simulink library "TOWER_MASTER"  (Simulink 8.8)
settings: Solver=ode45  StartTime=0.0  StopTime=10.0  RelTol=1e-3  EnableMultiTasking=on
undefined symbols (not defined in the file): AC, AC2THRESHOLD, BF_WD_MASTER, GAS_WD_MASTER, GASAC, SIXOSEM_F_WD_AC_MASTER
libraries: cdsEpicsOut x163, cdsFilt x111, cdsTP x68, cdsFiltCtrl x56, cdsEpicsIn x47, cdsMuxMatrix x14, cdsRms x14, TOWER_MASTER x11, STATE_BIO_MASTER x8, cdsEpicsBinIn x6, cdsFunctionCall x4, VIS_LIB x2
(part 16 of 19)

== system TOWER_MASTER/common_blocks/GASMASTER/SEISFF ==
  note: 1 (one) if GOOD
      | 0 (zero) if BAD
  note: Each DAMP filter output bitword is
      | compared against a known good state.
      | If equal to good state, then a 1 is output
      | and multiplied into the product. So, if any DOF
      | is not in its good state, the whole product is 0.
  SEIS_In : Inport
  GAS : cdsFiltCtrl/IIR FM with control  Tag=cdsFiltCtrl  Description=|
      | cdsFiltCntrl is the standard IIR filter module (exactly the same as cdsFilt) but with added control data output 'Ctrl'. Filter module digital signal output appears on the first output, which is called 'Val'. 'Ctrl' output has a bit pattern encoding the state of filter's on/off switches (FM1 through FM10). The bit values are:
      |                                                                                                                                                                                                                                                                                                                                       
      | module 	hex	dec                                                                                                                                                                                                                                                                                                                       
      | -----------------------                                                                                                                                                                                                                                                                                                               
      | FM1	0x20                    32                                                                                                                                                                                                                                                                                                        
      | FM2	0x80                     128                                                                                                                                                                                                                                                                                                      
      | FM3	0x200                   512                                                                                                                                                                                                                                                                                                       
      | FM4	0x800                   2048                                                                                                                                                                                                                                                                                                      
      | FM5	0x2000                 8192                                                                                                                                                                                                                                                                                                       
      | FM6	0x8000                 32768                                                                                                                                                                                                                                                                                                      
      | FM7	0x20000                131072                                                                                                                                                                                                                                                                                                     
      | FM8	0x80000                 524288                                                                                                                                                                                                                                                                                                    
      | FM9	0x200000               2097152                                                                                                                                                                                                                                                                                                    
      | FM10	0x800000               8388608                                                                                                                                                                                                                                                                                                   
      |                                                                                                                                                                                                                                                                                                                                       
      | This bit data can be used to drive some other switches or it can be output using a binary I/O module.
      settings: AttributesFormatString=%<Tag>
  GAS_STATE_GOOD : cdsEpicsIn/Subsystem  Tag=cdsEpicsIn  Description=|
      | Purpose:                                                                              
      | Create an EPICS input channel connection to the FE realtime controls.                 
      |                                                                                       
      | Operation:                                                                            
      | Outputs value from an EPICS ai record. Value is floating point with a precision of 3..
      |                                                                                       
      | Usage:                                                                                
      | Name the part with the desired EPICS channel name.
      settings: AttributesFormatString=%<Tag>
  GAS_STATE_NOW : cdsEpicsOut/Subsystem  Tag=cdsEpicsOutput  Description=|
      | Purpose:                                          
      | Output a FE signal to an EPICS channel.           
      |                                                   
      | Operation:                                        
      | Takes input value and passes it to EPICS record.  
      |                                                   
      | Usage:                                            
      | Name the part with the desired EPICS rrecord name.
      settings: AttributesFormatString=%<Tag>
  Ground6 : Ground
  Ground8 : Ground
  Operator : RelationalOperator  Operator===  OutDataTypeStr=boolean  RndMeth=Nearest
  STATE_OK : cdsEpicsOut/Subsystem  Tag=cdsEpicsOutput  Description=|
      | Purpose:                                          
      | Output a FE signal to an EPICS channel.           
      |                                                   
      | Operation:                                        
      | Takes input value and passes it to EPICS record.  
      |                                                   
      | Usage:                                            
      | Name the part with the desired EPICS rrecord name.
      settings: AttributesFormatString=%<Tag>
  SEIS_Out : Outport
  SEIS_STATE_Out : Outport  Port=2
  wires:
  Operator/1 -> STATE_OK/1
  Ground8/1 -> GAS/3
  STATE_OK/1 -> SEIS_STATE_Out/1
  GAS_STATE_NOW/1 -> Operator/2
  GAS/2 -> GAS_STATE_NOW/1
  GAS_STATE_GOOD/1 -> Operator/1
  GAS/1 -> SEIS_Out/1
  SEIS_In/1 -> GAS/1
  Ground6/1 -> GAS/2

== system TOWER_MASTER/common_blocks/GASMASTER/SENSCORR ==
  SEIS_GAS_In : Inport
  GAS : cdsFilt/Subsystem  Tag=cdsFilt  Description=|
      | Purpose:                                                                                                                                                                                                                                  
      | Standard CDS IIR filter module.                                                                                                                                                                                                           
      |                                                                                                                                                                                                                                           
      | Operation:                                                                                                                                                                                                                                
      | Consists of 10 second order section IIR filters, plus a ramped gain stage. In FE code, also provides pre-defined test points and excitation channel inputs. The filter coefficients are defined in the LIGO system using the 'foton' tool.
      |                                                                                                                                                                                                                                           
      | Usage:                                                                                                                                                                                                                                    
      | Name the part with the desired filter module name.
      settings: AttributesFormatString=%<Tag>
  SC_GAS_Out : Outport
  wires:
  GAS/1 -> SC_GAS_Out/1
  SEIS_GAS_In/1 -> GAS/1

== system TOWER_MASTER/common_blocks/GASMASTER/SET ==
  GAS : cdsFilt/Subsystem  Tag=cdsFilt  Description=|
      | Purpose:                                                                                                                                                                                                                                  
      | Standard CDS IIR filter module.                                                                                                                                                                                                           
      |                                                                                                                                                                                                                                           
      | Operation:                                                                                                                                                                                                                                
      | Consists of 10 second order section IIR filters, plus a ramped gain stage. In FE code, also provides pre-defined test points and excitation channel inputs. The filter coefficients are defined in the LIGO system using the 'foton' tool.
      |                                                                                                                                                                                                                                           
      | Usage:                                                                                                                                                                                                                                    
      | Name the part with the desired filter module name.
      settings: AttributesFormatString=%<Tag>
  Ground1 : Ground
  Ground7 : Ground
  STATUS : cdsEpicsBinIn/Subsystem  Tag=cdsEpicsBinIn  Description=|
      | Purpose:                                                                            
      | Create an EPICS binary (0 or 1) input channel to the FE realtime controls.          
      |                                                                                     
      | Operation:                                                                          
      | Outputs value from an EPICS ai record. Value is binary input (bi Epics record type).
      |                                                                                     
      | Usage:                                                                              
      | Name the part with the desired EPICS channel name.
      settings: AttributesFormatString=%<Tag>
  GAS_Out : Outport
  wires:
  Ground7/1 -> STATUS/1
  Ground1/1 -> GAS/1
  GAS/1 -> GAS_Out/1

== system TOWER_MASTER/common_blocks/GASMASTER/SUMOUT ==
  GAS_In : Inport
  GAS : cdsFilt/Subsystem  Tag=cdsFilt  Description=|
      | Purpose:                                                                                                                                                                                                                                  
      | Standard CDS IIR filter module.                                                                                                                                                                                                           
      |                                                                                                                                                                                                                                           
      | Operation:                                                                                                                                                                                                                                
      | Consists of 10 second order section IIR filters, plus a ramped gain stage. In FE code, also provides pre-defined test points and excitation channel inputs. The filter coefficients are defined in the LIGO system using the 'foton' tool.
      |                                                                                                                                                                                                                                           
      | Usage:                                                                                                                                                                                                                                    
      | Name the part with the desired filter module name.
      settings: AttributesFormatString=%<Tag>
  GAS_Out : Outport
  wires:
  GAS/1 -> GAS_Out/1
  GAS_In/1 -> GAS/1

== system TOWER_MASTER/common_blocks/GASMASTER/TEST ==
  GAS : cdsFilt/Subsystem  Tag=cdsFilt  Description=|
      | Purpose:                                                                                                                                                                                                                                  
      | Standard CDS IIR filter module.                                                                                                                                                                                                           
      |                                                                                                                                                                                                                                           
      | Operation:                                                                                                                                                                                                                                
      | Consists of 10 second order section IIR filters, plus a ramped gain stage. In FE code, also provides pre-defined test points and excitation channel inputs. The filter coefficients are defined in the LIGO system using the 'foton' tool.
      |                                                                                                                                                                                                                                           
      | Usage:                                                                                                                                                                                                                                    
      | Name the part with the desired filter module name.
      settings: AttributesFormatString=%<Tag>
  Ground1 : Ground
  Ground7 : Ground
  STATUS : cdsEpicsBinIn/Subsystem  Tag=cdsEpicsBinIn  Description=|
      | Purpose:                                                                            
      | Create an EPICS binary (0 or 1) input channel to the FE realtime controls.          
      |                                                                                     
      | Operation:                                                                          
      | Outputs value from an EPICS ai record. Value is binary input (bi Epics record type).
      |                                                                                     
      | Usage:                                                                              
      | Name the part with the desired EPICS channel name.
      settings: AttributesFormatString=%<Tag>
  GAS_Out : Outport
  wires:
  GAS/1 -> GAS_Out/1
  Ground1/1 -> GAS/1
  Ground7/1 -> STATUS/1

== system TOWER_MASTER/common_blocks/GASMASTER/WD ==
  GAS_In : Inport
  AC : Subsystem  AncestorBlock=GAS_WD_MASTER/GASAC
  GAS_AC_FLAG_Out : Outport
  wires:
  AC/1(FLAG) -> GAS_AC_FLAG_Out/1
  GAS_In/1 -> AC/1(H1_In)

== system TOWER_MASTER/common_blocks/OKUTOMIGASMODAL/ADD ==
  TEST_M1_In : Inport
  TEST_M2_In : Inport  Port=2
  TEST_M3_In : Inport  Port=3
  TEST_M4_In : Inport  Port=4
  TEST_M5_In : Inport  Port=5
  DAMP_M1_In : Inport  Port=6
  DAMP_M2_In : Inport  Port=7
  DAMP_M3_In : Inport  Port=8
  DAMP_M4_In : Inport  Port=9
  DAMP_M5_In : Inport  Port=10
  Sum{1..5} (5 alike) : Sum
  M1_MAIN_Out : Outport
  M2_MAIN_Out : Outport  Port=2
  M3_MAIN_Out : Outport  Port=3
  M4_MAIN_Out : Outport  Port=4
  M5_MAIN_Out : Outport  Port=5
  wires:
  DAMP_M5_In/1 -> Sum5/2
  TEST_M5_In/1 -> Sum5/1
  Sum5/1 -> M5_MAIN_Out/1
  DAMP_M4_In/1 -> Sum4/2
  TEST_M4_In/1 -> Sum4/1
  DAMP_M3_In/1 -> Sum3/2
  TEST_M3_In/1 -> Sum3/1
  DAMP_M2_In/1 -> Sum2/2
  TEST_M2_In/1 -> Sum2/1
  TEST_M1_In/1 -> Sum1/1
  DAMP_M1_In/1 -> Sum1/2
  Sum3/1 -> M3_MAIN_Out/1
  Sum4/1 -> M4_MAIN_Out/1
  Sum1/1 -> M1_MAIN_Out/1
  Sum2/1 -> M2_MAIN_Out/1
